simulink model "Copy_of_LQR_lp1_1"  (R2021a)
settings: Solver=ode4  StartTime=0.0  StopTime=inf  FixedStep=0.001  RelTol=1e-3
libraries: ETlabLibrary x5
settings Model: SimulationMode=external  Creator=Administrator  LastModifiedBy=YW
settings SolverCC: AlgebraicLoopSolver=TrustRegion  DecoupledContinuousIntegration=on  MinimalZcImpactIntegration=on
settings DataIOCC: ReturnWorkspaceOutputs=off
settings DebuggingCC: SFMachineParentedDataDiag=warning  ArithmeticOperatorsInVariantConditions=warning
settings SFSimCC: SimUseLocalCustomCode=off  CustomCodeUndefinedFunction=UseInterfaceOnly
settings RTWCC: Description=Simulink Desktop Real-Time  SystemTargetFile=sldrt.tlc  TemplateMakefile=sldrt.tmf  RTWUseLocalCustomCode=off  RTWCompilerOptimization=on
settings CodeAppCC: MaxIdLength=95
settings SimulinkDesktopRealTimeCC: TargetPreCompLibLocation=D:\matlab2021a\toolbox\sldrt\lib\win64

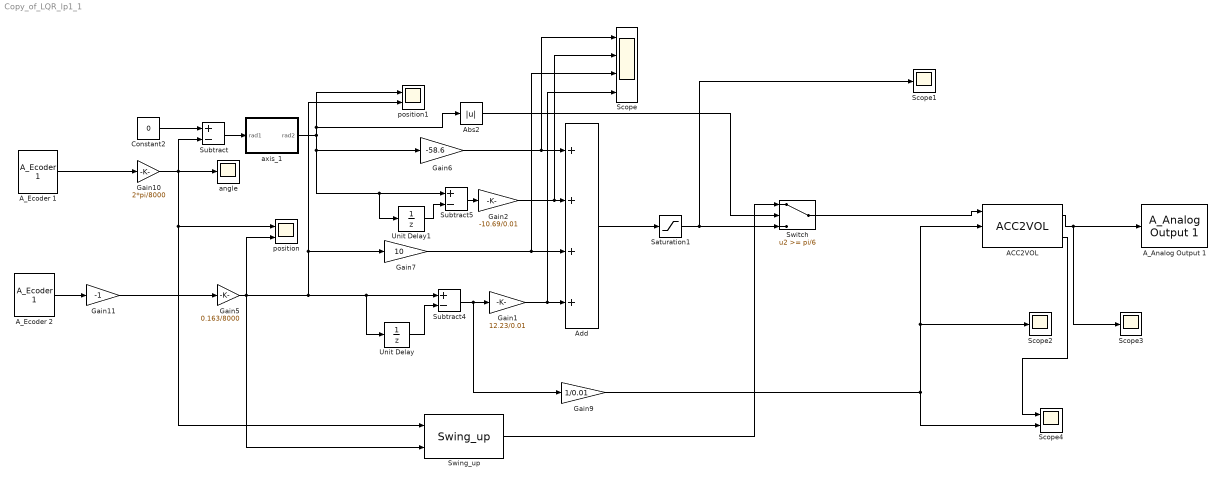
== system Copy_of_LQR_lp1_1 ==
  ACC2VOL : ETlabLibrary/ACC2VOL  PGain=0.18  IGain=54  VelocityUpper=0.6  VelocityLower=-0.6  VoltageUpper=1  VoltageLower=-1  Ts=0.005
      settings: SourceProductName=ETlabLibrary
  A_Analog Output 1 : ETlabLibrary/A_Analog Output 1  SampleTime=0.01
      settings: SourceProductName=ETlabLibrary
  A_Ecoder 1 : ETlabLibrary/A_Ecoder 1  SampleTime=0.01
      link override Encoder 01: SampleTime=SampleTime  MaxMissedTicks=10000000000000000000  ShowMissedTicks=off  YieldWhenWaiting=on  DrvName=National_Instruments/PCI-6602  DrvAddress=4294967295  DrvOptions=[0 2 2 2 2 0 0 0 0]  Channels=2  QuadMode=3  IndexPulse=1  InputFilter=Inf  DataType=1
      settings: SourceProductName=ETlabLibrary
  A_Ecoder 2 : ETlabLibrary/A_Ecoder 1  SampleTime=0.01
      link override Encoder 01: SampleTime=SampleTime  MaxMissedTicks=10000000  ShowMissedTicks=off  YieldWhenWaiting=on  DrvName=National_Instruments/PCI-6602  DrvAddress=4294967295  DrvOptions=[0 0 0 0 0 0 0 0 0]  Channels=1  QuadMode=3  IndexPulse=1  InputFilter=Inf  DataType=1
      link override Encoder Input4: SampleTime=SampleTime  MaxMissedTicks=1000000  ShowMissedTicks=off  YieldWhenWaiting=off  DrvName=National_Instruments/PCI-6602  DrvAddress=4294967295  DrvOptions=[255 3 3 3 2 2 2 2 2]  Channels=5  QuadMode=3  IndexPulse=2  InputFilter=Inf  DataType=1
      settings: SourceProductName=ETlabLibrary
  Abs2 : Abs
  Add : Sum  Inputs=++++
  Constant2 : Constant  Value=0
  Gain1 : Gain  Gain=12.23/0.01  OutDataTypeStr=double
  Gain10 : Gain  Gain=2*pi/8000  OutDataTypeStr=double
  Gain11 : Gain  Gain=-1  OutDataTypeStr=double
  Gain2 : Gain  Gain=-10.69/0.01  OutDataTypeStr=double
  Gain5 : Gain  Gain=0.163/8000  OutDataTypeStr=double
  Gain6 : Gain  Gain=-58.6  OutDataTypeStr=double
  Gain7 : Gain  Gain=10  OutDataTypeStr=double
  Gain9 : Gain  Gain=1/0.01  OutDataTypeStr=double
  Saturation1 : Saturate  UpperLimit=10  LowerLimit=-10
  Scope : Scope  NumInputPorts=4
  Scope1 : Scope
  Scope2 : Scope
  Scope3 : Scope
  Scope4 : Scope  NumInputPorts=2
  Subtract : Sum  Inputs=+-
  Subtract4 : Sum  Inputs=+-
  Subtract5 : Sum  Inputs=+-
  Swing_up : ETlabLibrary/Swing_up  m=0.134  g=9.8  l=0.223  J=0.0089  AccUpper=10  AccLower=-10  Gain1=5  Gain2=6  PositionLimit=0.25  Ts=0.01
      settings: SourceProductName=ETlabLibrary
  Switch : Switch  Threshold=pi/6
  Unit Delay : UnitDelay  SampleTime=0.01  HasFrameUpgradeWarning=on
  Unit Delay1 : UnitDelay  SampleTime=0.01  HasFrameUpgradeWarning=on
  angle : Scope
  axis_1 : MATLAB Function  TreatAsAtomicUnit=on
  position : Scope  NumInputPorts=2
  position1 : Scope  NumInputPorts=2
  wires:
  Gain1/1 -> Add/4, Scope/4
  Gain2/1 -> Scope/2, Add/2
  Constant2/1 -> Subtract/1
  Subtract/1 -> axis_1/1(rad1)
  Gain6/1 -> Scope/1, Add/1
  Gain7/1 -> Scope/3, Add/3
  Gain10/1 -> Swing_up/1, position/1, angle/1, Subtract/2
  Abs2/1 -> Switch/2
  Subtract4/1 -> Gain9/1, Gain1/1
  Gain5/1 -> Swing_up/2, position/2, Unit Delay/1, Subtract4/1, Gain7/1, position1/2
  Unit Delay/1 -> Subtract4/2
  Subtract5/1 -> Gain2/1
  axis_1/1(rad2) -> Subtract5/1, Unit Delay1/1, Gain6/1, position1/1, Abs2/1
  Unit Delay1/1 -> Subtract5/2
  A_Ecoder 2/1 -> Gain11/1
  A_Ecoder 1/1 -> Gain10/1
  Gain11/1 -> Gain5/1
  Add/1 -> Saturation1/1
  Saturation1/1 -> Scope1/1, Switch/3
  Switch/1 -> ACC2VOL/1
  Gain9/1 -> Scope2/1, ACC2VOL/2, Scope4/2
  Swing_up/1 -> Switch/1
  ACC2VOL/2 -> Scope4/1
  ACC2VOL/1 -> A_Analog Output 1/1, Scope3/1

== matlab function Copy_of_LQR_lp1_1/axis_1 ==
  data: rad1 input; rad2 output
function rad2 = ChangeRad(rad1)

while(rad1>pi)
    rad1 = rad1 - 2 * pi;
end
while(rad1<-pi)
    rad1 = rad1 + 2 * pi;
end

rad2 = rad1;
